simulink model "Simulink_Ivezic_2x2"  (R2021a)
settings: Solver=ode45  StartTime=0.0  StopTime=10000  RelTol=1e-3
model workspace (MAT data in the model file):
  Gm = tf
  Gm.IOSize_ = [2 2]
  Gm.Data_ = ltipack.tfdata
  Gm.Data_.num = {[0 87.8], [0 -86.4]; [0 108.2], [0 -109.6]}
  Gm.Data_.den = {[75 1], [75 1]; [75 1], [75 1]}
  Gm.Data_.Delay.Input = [0; 0]
  Gm.Data_.Delay.Output = [0; 0]
  Gm.Data_.Delay.IO = [0  0; 0  0]
  Gm.Data_.Ts = 0
undefined symbols (not defined in the file or in its folder): D, Did, Dstatic, G, kck_1, kck_2, kd_1, kd_2, ki_1, ki_2, Tdio
libraries: cstextras x12, pid_lib x4
Description:
  | The LTISystemBlockMIMO model shows how to use an LTI System block to represent a MIMO plant in a control system.
settings Model: Creator=The MathWorks, Inc.  LastModifiedBy=Grazielle
settings SolverCC: AlgebraicLoopSolver=LineSearch
settings DataIOCC: ReturnWorkspaceOutputs=off
settings DebuggingCC: SFMachineParentedDataDiag=warning  ArithmeticOperatorsInVariantConditions=warning
settings SFSimCC: SimUseLocalCustomCode=off  CustomCodeUndefinedFunction=UseInterfaceOnly
settings RTWCC: RTWUseLocalCustomCode=off
settings CodeAppCC: StateflowObjectComments=on
settings ConfigComp: CovMetricSettings=dswe

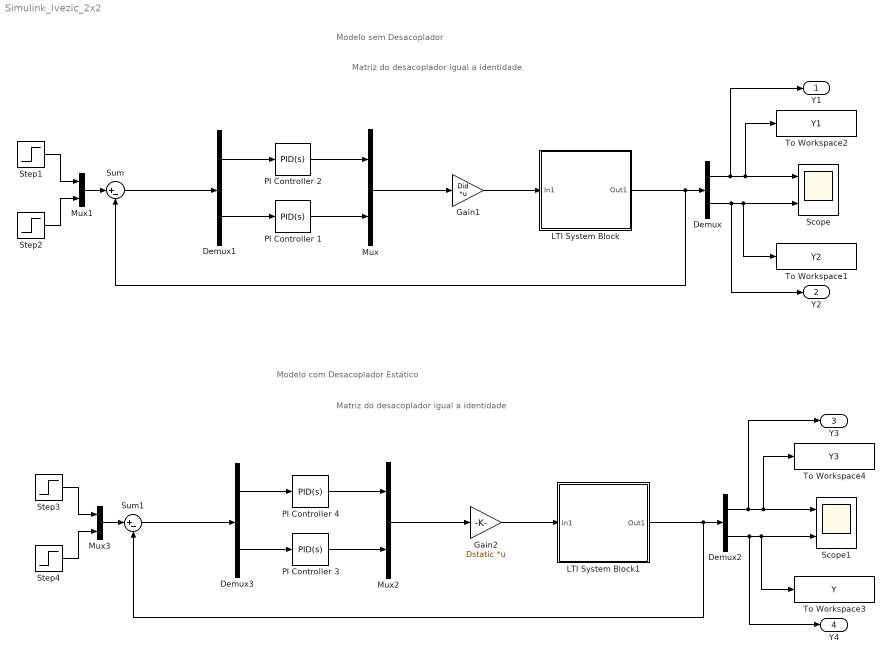
== system Simulink_Ivezic_2x2 ==
  note: Matriz do desacoplador igual a identidade
  note: Modelo sem Desacoplador
  note: Matriz do desacoplador igual a identidade
  note: Modelo com Desacoplador Estático
  Demux{,1..3} (4 alike) : Demux  Outputs=2
  Gain1 : Gain  Gain=Did  Multiplication=Matrix(K*u)
  Gain2 : Gain  Gain=Dstatic  Multiplication=Matrix(K*u)
  LTI System Block : Subsystem  AncestorBlock=cstblocks/LTI System  BlockChoice=CSS  mask(LTI Block){sys=G, IC=[]}
      mask prompts: sys "Control:simulink:LTIMaskLabel1"; IC "Control:simulink:LTIMaskLabel2"
      mask help: Control:simulink:LTIMaskDescription
      mask init:
      | try
      |    % read data to initialize mask variables
      |    [D,Ts,Tdi,Tdo,Tdio,x0,sysname]=...
      |       ltimask('Initialize',gcb,sys,IC);
      |    % update contents
      |    model = bdroot;
      |    df = get_param(model,'dirty');
      |    ltimask('UpdateDiagram',gcb,D,Ts,Tdio);
      |    try      
      |       % Attempt to modify locked library -> error
      |       % Makes block show ??? when loading CSTBLOCKS
      |       % for the first time
      |       set_param(model,'dirty',df)
      |    end
      | catch ME
      |    sys = [];  IC = [];   sysname = '???';
      |    throw(ME)
      | end
      mask Help: eval('ctrlguihelp(''ltisystemblock'');')
      mask Callback sys: ltimask('MaskLTICallback',gcb);
      mask DialogControl sys Prompt: LTI system variable
      mask DialogControl IC Prompt: Initial states (state-space only)
      mask Display: disp(sysname)
  LTI System Block1 : Subsystem  AncestorBlock=cstblocks/LTI System  BlockChoice=CSS  mask(LTI Block){sys=G, IC=[]}
      mask prompts: sys "Control:simulink:LTIMaskLabel1"; IC "Control:simulink:LTIMaskLabel2"
      mask help: Control:simulink:LTIMaskDescription
      mask init: same as Simulink_Ivezic_2x2/LTI System Block
      mask Help: eval('ctrlguihelp(''ltisystemblock'');')
      mask Callback sys: ltimask('MaskLTICallback',gcb);
      mask DialogControl sys Prompt: LTI system variable
      mask DialogControl IC Prompt: Initial states (state-space only)
      mask Display: disp(sysname)
  Mux{,1..3} (4 alike) : Mux  Inputs=2
  PI Controller 1 : pid_lib/PID Controller  Controller=PID  Form=Parallel  TimeDomain=Continuous-time  UseExternalTs=off  SampleTime=-1  IntegratorMethod=Forward Euler  FilterMethod=Forward Euler  ControllerParametersSource=internal  P=kck_2  I=ki_2  D=kd_2  UseFilter=on  N=0  TunerSelectOption=Transfer Function Based (PID Tuner App)  InitialConditionSource=internal  InitialConditionForIntegrator=0  InitialConditionForFilter=0  DifferentiatorICPrevScaledInput=0  ExternalReset=none  TrackingMode=off  Kt=1  LimitOutput=off  SatLimitsSource=internal  UpperSaturationLimit=inf  LowerSaturationLimit=-inf  LinearizeAsGain=on  AntiWindupMode=none  Kb=1  POutMin=[]  POutMax=[]  IOutMin=[]  IOutMax=[]  DOutMin=[]  DOutMax=[]  NOutMin=[]  NOutMax=[]  SumOutMin=[]  SumOutMax=[]  SaturationOutMin=[]  SaturationOutMax=[]  PParamMin=[]  PParamMax=[]  IParamMin=[]  IParamMax=[]  DParamMin=[]  DParamMax=[]  NParamMin=[]  NParamMax=[]  KbParamMin=[]  KbParamMax=[]  KtParamMin=[]  KtParamMax=[]  KbOutMin=[]  KbOutMax=[]  KtOutMin=[]  KtOutMax=[]  IntegratorOutMin=[]  IntegratorOutMax=[]  FilterOutMin=[]  FilterOutMax=[]  SumI1OutMin=[]  SumI1OutMax=[]  SumI2OutMin=[]  SumI2OutMax=[]  SumI3OutMin=[]  SumI3OutMax=[]  SumI4OutMin=[]  SumI4OutMax=[]  SumDOutMin=[]  SumDOutMax=[]  DifferentiatorOutMin=[]  DifferentiatorOutMax=[]  FilterDiffOutCoefMin=[]  FilterDiffOutCoefMax=[]  ReciprocalOutMin=[]  ReciprocalOutMax=[]  SumDenOutMin=[]  SumDenOutMax=[]  SumNumOutMin=[]  SumNumOutMax=[]  DivideOutMin=[]  DivideOutMax=[]  UdiffTsProdOutMin=[]  UdiffTsProdOutMax=[]  NTsProdOutMin=[]  NTsProdOutMax=[]  UintegralTsProdOutMin=[]  UintegralTsProdOutMax=[]  UngainTsProdOutMin=[]  UngainTsProdOutMax=[]  IntegratorContinuousStateAttributes=''  IntegratorStateMustResolveToSignalObject=off  IntegratorRTWStateStorageClass=Auto  FilterContinuousStateAttributes=''  FilterStateMustResolveToSignalObject=off  FilterRTWStateStorageClass=Auto  ParallelPVariant=InternalParameters  IdealPVariant=Disabled  IVariant=InternalParameters  DVariant=InternalParameters  IntegratorVariant=Continuous  SatVariant=Disabled  AWVariant=Passthrough  PCopyVariant=Disabled  TRVariant=Disabled  FdbkBlocksVariant=Forward  IdealPFdbkVariant=Disabled  SatFdbkVariant=Disabled  DerivativeFilterVariant=ContFilter  NVariant=InternalParameters  NCopyVariant=Disabled  FilterICVariant=InternalICsFilter  IntegratorICVariant=InternalICs  ExternalResetVariant=Disabled  TRSumVariant=Passthrough  SumFdbkVariant=Disabled  SumVariant=Sum_PID  TsampFilterVariant=InternalTs  TsampNgainVariant=Passthrough  TsampIntegralVariant=Passthrough  ExternalSaturationOutDataTypeStr=Inherit: Same as second input
  PI Controller 2 : pid_lib/PID Controller  Controller=PID  Form=Parallel  TimeDomain=Continuous-time  UseExternalTs=off  SampleTime=-1  IntegratorMethod=Forward Euler  FilterMethod=Forward Euler  ControllerParametersSource=internal  P=kck_1  I=ki_1  D=kd_1  UseFilter=on  N=0  TunerSelectOption=Transfer Function Based (PID Tuner App)  InitialConditionSource=internal  InitialConditionForIntegrator=0  InitialConditionForFilter=0  DifferentiatorICPrevScaledInput=0  ExternalReset=none  TrackingMode=off  Kt=1  LimitOutput=off  SatLimitsSource=internal  UpperSaturationLimit=inf  LowerSaturationLimit=-inf  LinearizeAsGain=on  AntiWindupMode=none  Kb=1  POutMin=[]  POutMax=[]  IOutMin=[]  IOutMax=[]  DOutMin=[]  DOutMax=[]  NOutMin=[]  NOutMax=[]  SumOutMin=[]  SumOutMax=[]  SaturationOutMin=[]  SaturationOutMax=[]  PParamMin=[]  PParamMax=[]  IParamMin=[]  IParamMax=[]  DParamMin=[]  DParamMax=[]  NParamMin=[]  NParamMax=[]  KbParamMin=[]  KbParamMax=[]  KtParamMin=[]  KtParamMax=[]  KbOutMin=[]  KbOutMax=[]  KtOutMin=[]  KtOutMax=[]  IntegratorOutMin=[]  IntegratorOutMax=[]  FilterOutMin=[]  FilterOutMax=[]  SumI1OutMin=[]  SumI1OutMax=[]  SumI2OutMin=[]  SumI2OutMax=[]  SumI3OutMin=[]  SumI3OutMax=[]  SumI4OutMin=[]  SumI4OutMax=[]  SumDOutMin=[]  SumDOutMax=[]  DifferentiatorOutMin=[]  DifferentiatorOutMax=[]  FilterDiffOutCoefMin=[]  FilterDiffOutCoefMax=[]  ReciprocalOutMin=[]  ReciprocalOutMax=[]  SumDenOutMin=[]  SumDenOutMax=[]  SumNumOutMin=[]  SumNumOutMax=[]  DivideOutMin=[]  DivideOutMax=[]  UdiffTsProdOutMin=[]  UdiffTsProdOutMax=[]  NTsProdOutMin=[]  NTsProdOutMax=[]  UintegralTsProdOutMin=[]  UintegralTsProdOutMax=[]  UngainTsProdOutMin=[]  UngainTsProdOutMax=[]  IntegratorContinuousStateAttributes=''  IntegratorStateMustResolveToSignalObject=off  IntegratorRTWStateStorageClass=Auto  FilterContinuousStateAttributes=''  FilterStateMustResolveToSignalObject=off  FilterRTWStateStorageClass=Auto  ParallelPVariant=InternalParameters  IdealPVariant=Disabled  IVariant=InternalParameters  DVariant=InternalParameters  IntegratorVariant=Continuous  SatVariant=Disabled  AWVariant=Passthrough  PCopyVariant=Disabled  TRVariant=Disabled  FdbkBlocksVariant=Forward  IdealPFdbkVariant=Disabled  SatFdbkVariant=Disabled  DerivativeFilterVariant=ContFilter  NVariant=InternalParameters  NCopyVariant=Disabled  FilterICVariant=InternalICsFilter  IntegratorICVariant=InternalICs  ExternalResetVariant=Disabled  TRSumVariant=Passthrough  SumFdbkVariant=Disabled  SumVariant=Sum_PID  TsampFilterVariant=InternalTs  TsampNgainVariant=Passthrough  TsampIntegralVariant=Passthrough  ExternalSaturationOutDataTypeStr=Inherit: Same as second input
  PI Controller 3 : pid_lib/PID Controller  Controller=PID  Form=Parallel  TimeDomain=Continuous-time  UseExternalTs=off  SampleTime=-1  IntegratorMethod=Forward Euler  FilterMethod=Forward Euler  ControllerParametersSource=internal  P=kck_2  I=ki_2  D=kd_2  UseFilter=on  N=0  TunerSelectOption=Transfer Function Based (PID Tuner App)  InitialConditionSource=internal  InitialConditionForIntegrator=0  InitialConditionForFilter=0  DifferentiatorICPrevScaledInput=0  ExternalReset=none  TrackingMode=off  Kt=1  LimitOutput=off  SatLimitsSource=internal  UpperSaturationLimit=inf  LowerSaturationLimit=-inf  LinearizeAsGain=on  AntiWindupMode=none  Kb=1  POutMin=[]  POutMax=[]  IOutMin=[]  IOutMax=[]  DOutMin=[]  DOutMax=[]  NOutMin=[]  NOutMax=[]  SumOutMin=[]  SumOutMax=[]  SaturationOutMin=[]  SaturationOutMax=[]  PParamMin=[]  PParamMax=[]  IParamMin=[]  IParamMax=[]  DParamMin=[]  DParamMax=[]  NParamMin=[]  NParamMax=[]  KbParamMin=[]  KbParamMax=[]  KtParamMin=[]  KtParamMax=[]  KbOutMin=[]  KbOutMax=[]  KtOutMin=[]  KtOutMax=[]  IntegratorOutMin=[]  IntegratorOutMax=[]  FilterOutMin=[]  FilterOutMax=[]  SumI1OutMin=[]  SumI1OutMax=[]  SumI2OutMin=[]  SumI2OutMax=[]  SumI3OutMin=[]  SumI3OutMax=[]  SumI4OutMin=[]  SumI4OutMax=[]  SumDOutMin=[]  SumDOutMax=[]  DifferentiatorOutMin=[]  DifferentiatorOutMax=[]  FilterDiffOutCoefMin=[]  FilterDiffOutCoefMax=[]  ReciprocalOutMin=[]  ReciprocalOutMax=[]  SumDenOutMin=[]  SumDenOutMax=[]  SumNumOutMin=[]  SumNumOutMax=[]  DivideOutMin=[]  DivideOutMax=[]  UdiffTsProdOutMin=[]  UdiffTsProdOutMax=[]  NTsProdOutMin=[]  NTsProdOutMax=[]  UintegralTsProdOutMin=[]  UintegralTsProdOutMax=[]  UngainTsProdOutMin=[]  UngainTsProdOutMax=[]  IntegratorContinuousStateAttributes=''  IntegratorStateMustResolveToSignalObject=off  IntegratorRTWStateStorageClass=Auto  FilterContinuousStateAttributes=''  FilterStateMustResolveToSignalObject=off  FilterRTWStateStorageClass=Auto  ParallelPVariant=InternalParameters  IdealPVariant=Disabled  IVariant=InternalParameters  DVariant=InternalParameters  IntegratorVariant=Continuous  SatVariant=Disabled  AWVariant=Passthrough  PCopyVariant=Disabled  TRVariant=Disabled  FdbkBlocksVariant=Forward  IdealPFdbkVariant=Disabled  SatFdbkVariant=Disabled  DerivativeFilterVariant=ContFilter  NVariant=InternalParameters  NCopyVariant=Disabled  FilterICVariant=InternalICsFilter  IntegratorICVariant=InternalICs  ExternalResetVariant=Disabled  TRSumVariant=Passthrough  SumFdbkVariant=Disabled  SumVariant=Sum_PID  TsampFilterVariant=InternalTs  TsampNgainVariant=Passthrough  TsampIntegralVariant=Passthrough  ExternalSaturationOutDataTypeStr=Inherit: Same as second input
  PI Controller 4 : pid_lib/PID Controller  Controller=PID  Form=Parallel  TimeDomain=Continuous-time  UseExternalTs=off  SampleTime=-1  IntegratorMethod=Forward Euler  FilterMethod=Forward Euler  ControllerParametersSource=internal  P=kck_1  I=ki_1  D=kd_1  UseFilter=on  N=0  TunerSelectOption=Transfer Function Based (PID Tuner App)  InitialConditionSource=internal  InitialConditionForIntegrator=0  InitialConditionForFilter=0  DifferentiatorICPrevScaledInput=0  ExternalReset=none  TrackingMode=off  Kt=1  LimitOutput=off  SatLimitsSource=internal  UpperSaturationLimit=inf  LowerSaturationLimit=-inf  LinearizeAsGain=on  AntiWindupMode=none  Kb=1  POutMin=[]  POutMax=[]  IOutMin=[]  IOutMax=[]  DOutMin=[]  DOutMax=[]  NOutMin=[]  NOutMax=[]  SumOutMin=[]  SumOutMax=[]  SaturationOutMin=[]  SaturationOutMax=[]  PParamMin=[]  PParamMax=[]  IParamMin=[]  IParamMax=[]  DParamMin=[]  DParamMax=[]  NParamMin=[]  NParamMax=[]  KbParamMin=[]  KbParamMax=[]  KtParamMin=[]  KtParamMax=[]  KbOutMin=[]  KbOutMax=[]  KtOutMin=[]  KtOutMax=[]  IntegratorOutMin=[]  IntegratorOutMax=[]  FilterOutMin=[]  FilterOutMax=[]  SumI1OutMin=[]  SumI1OutMax=[]  SumI2OutMin=[]  SumI2OutMax=[]  SumI3OutMin=[]  SumI3OutMax=[]  SumI4OutMin=[]  SumI4OutMax=[]  SumDOutMin=[]  SumDOutMax=[]  DifferentiatorOutMin=[]  DifferentiatorOutMax=[]  FilterDiffOutCoefMin=[]  FilterDiffOutCoefMax=[]  ReciprocalOutMin=[]  ReciprocalOutMax=[]  SumDenOutMin=[]  SumDenOutMax=[]  SumNumOutMin=[]  SumNumOutMax=[]  DivideOutMin=[]  DivideOutMax=[]  UdiffTsProdOutMin=[]  UdiffTsProdOutMax=[]  NTsProdOutMin=[]  NTsProdOutMax=[]  UintegralTsProdOutMin=[]  UintegralTsProdOutMax=[]  UngainTsProdOutMin=[]  UngainTsProdOutMax=[]  IntegratorContinuousStateAttributes=''  IntegratorStateMustResolveToSignalObject=off  IntegratorRTWStateStorageClass=Auto  FilterContinuousStateAttributes=''  FilterStateMustResolveToSignalObject=off  FilterRTWStateStorageClass=Auto  ParallelPVariant=InternalParameters  IdealPVariant=Disabled  IVariant=InternalParameters  DVariant=InternalParameters  IntegratorVariant=Continuous  SatVariant=Disabled  AWVariant=Passthrough  PCopyVariant=Disabled  TRVariant=Disabled  FdbkBlocksVariant=Forward  IdealPFdbkVariant=Disabled  SatFdbkVariant=Disabled  DerivativeFilterVariant=ContFilter  NVariant=InternalParameters  NCopyVariant=Disabled  FilterICVariant=InternalICsFilter  IntegratorICVariant=InternalICs  ExternalResetVariant=Disabled  TRSumVariant=Passthrough  SumFdbkVariant=Disabled  SumVariant=Sum_PID  TsampFilterVariant=InternalTs  TsampNgainVariant=Passthrough  TsampIntegralVariant=Passthrough  ExternalSaturationOutDataTypeStr=Inherit: Same as second input
  Scope : Scope  NumInputPorts=2
  Scope1 : Scope  NumInputPorts=2
  Step{1..4} (4 alike) : Step  SampleTime=0
  Sum : Sum  Inputs=|+-
  Sum1 : Sum  Inputs=|+-
  To Workspace1 : ToWorkspace  VariableName=Y2  SaveFormat=Timeseries  SampleTime=-1
  To Workspace2 : ToWorkspace  VariableName=Y1  SaveFormat=Timeseries  SampleTime=-1
  To Workspace3 : ToWorkspace  VariableName=Y  SaveFormat=Timeseries  SampleTime=-1
  To Workspace4 : ToWorkspace  VariableName=Y3  SaveFormat=Timeseries  SampleTime=-1
  Y1 : Outport
  Y2 : Outport  Port=2
  Y3 : Outport  Port=3
  Y4 : Outport  Port=4
  wires:
  Demux/1 -> Y1/1, To Workspace2/1, Scope/1
  PI Controller 1/1 -> Mux/2
  PI Controller 2/1 -> Mux/1
  Sum/1 -> Demux1/1
  Demux1/1 -> PI Controller 2/1
  Demux1/2 -> PI Controller 1/1
  Step1/1 -> Mux1/1
  Step2/1 -> Mux1/2
  LTI System Block/1(Out1) -> Sum/2, Demux/1
  Mux1/1 -> Sum/1
  Mux/1 -> Gain1/1
  Gain1/1 -> LTI System Block/1(In1)
  Demux/2 -> Y2/1, To Workspace1/1, Scope/2
  Gain2/1 -> LTI System Block1/1(In1)
  Demux3/1 -> PI Controller 4/1
  Step4/1 -> Mux3/2
  Mux3/1 -> Sum1/1
  Demux2/2 -> Y4/1, To Workspace3/1, Scope1/2
  Mux2/1 -> Gain2/1
  LTI System Block1/1(Out1) -> Sum1/2, Demux2/1
  PI Controller 4/1 -> Mux2/1
  Step3/1 -> Mux3/1
  PI Controller 3/1 -> Mux2/2
  Demux3/2 -> PI Controller 3/1
  Sum1/1 -> Demux3/1
  Demux2/1 -> Y3/1, To Workspace4/1, Scope1/1

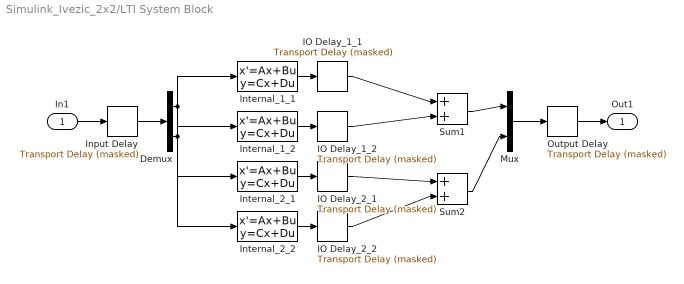
== system Simulink_Ivezic_2x2/LTI System Block ==
  In1 : Inport
  Demux : Demux  Outputs=2
  IO Delay_1_1 : cstextras/Transport Delay (masked)  Td=Tdio(1,1)  u0=0  bufsize=1024
      settings: SourceProductBaseCode=CT
  IO Delay_1_2 : cstextras/Transport Delay (masked)  Td=Tdio(1,2)  u0=0  bufsize=1024
      settings: SourceProductBaseCode=CT
  IO Delay_2_1 : cstextras/Transport Delay (masked)  Td=Tdio(2,1)  u0=0  bufsize=1024
      settings: SourceProductBaseCode=CT
  IO Delay_2_2 : cstextras/Transport Delay (masked)  Td=Tdio(2,2)  u0=0  bufsize=1024
      settings: SourceProductBaseCode=CT
  Input Delay : cstextras/Transport Delay (masked)  Td=Tdi  u0=0  bufsize=1024
      settings: SourceProductBaseCode=CT
  Internal_1_1 : StateSpace  A=D(1,1).a  B=D(1,1).b  C=D(1,1).c  D=D(1,1).d
  Internal_1_2 : StateSpace  A=D(1,2).a  B=D(1,2).b  C=D(1,2).c  D=D(1,2).d
  Internal_2_1 : StateSpace  A=D(2,1).a  B=D(2,1).b  C=D(2,1).c  D=D(2,1).d
  Internal_2_2 : StateSpace  A=D(2,2).a  B=D(2,2).b  C=D(2,2).c  D=D(2,2).d
  Mux : Mux  Inputs=2
  Output Delay : cstextras/Transport Delay (masked)  Td=Tdo  u0=0  bufsize=1024
      settings: SourceProductBaseCode=CT
  Sum1 : Sum
  Sum2 : Sum
  Out1 : Outport  InitialOutput=0  VectorParamsAs1DForOutWhenUnconnected=off
  wires:
  In1/1 -> Input Delay/1
  Output Delay/1 -> Out1/1
  Input Delay/1 -> Demux/1
  Mux/1 -> Output Delay/1
  Sum1/1 -> Mux/1
  Sum2/1 -> Mux/2
  Demux/1 -> Internal_1_1/1, Internal_2_1/1
  Internal_1_1/1 -> IO Delay_1_1/1
  IO Delay_1_1/1 -> Sum1/1
  Demux/2 -> Internal_1_2/1, Internal_2_2/1
  Internal_1_2/1 -> IO Delay_1_2/1
  IO Delay_1_2/1 -> Sum1/2
  Internal_2_1/1 -> IO Delay_2_1/1
  IO Delay_2_1/1 -> Sum2/1
  Internal_2_2/1 -> IO Delay_2_2/1
  IO Delay_2_2/1 -> Sum2/2

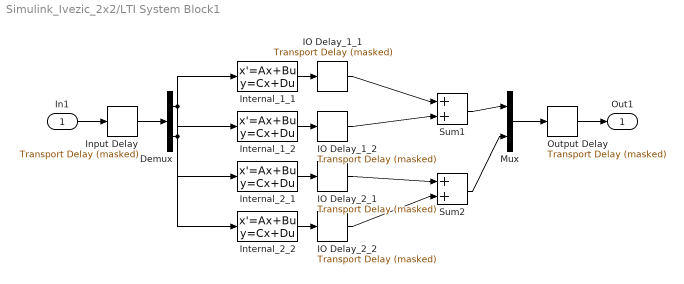
== system Simulink_Ivezic_2x2/LTI System Block1 ==
  In1 : Inport
  Demux : Demux  Outputs=2
  IO Delay_1_1 : cstextras/Transport Delay (masked)  Td=Tdio(1,1)  u0=0  bufsize=1024
      settings: SourceProductBaseCode=CT
  IO Delay_1_2 : cstextras/Transport Delay (masked)  Td=Tdio(1,2)  u0=0  bufsize=1024
      settings: SourceProductBaseCode=CT
  IO Delay_2_1 : cstextras/Transport Delay (masked)  Td=Tdio(2,1)  u0=0  bufsize=1024
      settings: SourceProductBaseCode=CT
  IO Delay_2_2 : cstextras/Transport Delay (masked)  Td=Tdio(2,2)  u0=0  bufsize=1024
      settings: SourceProductBaseCode=CT
  Input Delay : cstextras/Transport Delay (masked)  Td=Tdi  u0=0  bufsize=1024
      settings: SourceProductBaseCode=CT
  Internal_1_1 : StateSpace  A=D(1,1).a  B=D(1,1).b  C=D(1,1).c  D=D(1,1).d
  Internal_1_2 : StateSpace  A=D(1,2).a  B=D(1,2).b  C=D(1,2).c  D=D(1,2).d
  Internal_2_1 : StateSpace  A=D(2,1).a  B=D(2,1).b  C=D(2,1).c  D=D(2,1).d
  Internal_2_2 : StateSpace  A=D(2,2).a  B=D(2,2).b  C=D(2,2).c  D=D(2,2).d
  Mux : Mux  Inputs=2
  Output Delay : cstextras/Transport Delay (masked)  Td=Tdo  u0=0  bufsize=1024
      settings: SourceProductBaseCode=CT
  Sum1 : Sum
  Sum2 : Sum
  Out1 : Outport  InitialOutput=0  VectorParamsAs1DForOutWhenUnconnected=off
  wires:
  In1/1 -> Input Delay/1
  Output Delay/1 -> Out1/1
  Input Delay/1 -> Demux/1
  Mux/1 -> Output Delay/1
  Sum1/1 -> Mux/1
  Sum2/1 -> Mux/2
  Demux/1 -> Internal_1_1/1, Internal_2_1/1
  Internal_1_1/1 -> IO Delay_1_1/1
  IO Delay_1_1/1 -> Sum1/1
  Demux/2 -> Internal_1_2/1, Internal_2_2/1
  Internal_1_2/1 -> IO Delay_1_2/1
  IO Delay_1_2/1 -> Sum1/2
  Internal_2_1/1 -> IO Delay_2_1/1
  IO Delay_2_1/1 -> Sum2/1
  Internal_2_2/1 -> IO Delay_2_2/1
  IO Delay_2_2/1 -> Sum2/2
